simulink subsystem "joystick_to_pwm"  (R2025b)
settings: Solver=VariableStepAuto  StartTime=0.0  StopTime=10.0  RelTol=1e-3
settings Model: Creator=vulcangrip  LastModifiedBy=vulcangrip

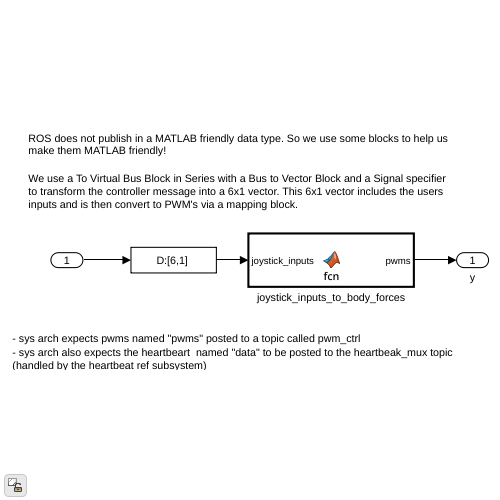
[thumbnail: Simulink's stored preview of the top-level diagram]
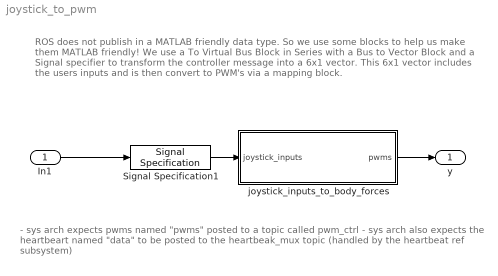
== system joystick_to_pwm ==
  note: - sys arch expects pwms named "pwms" posted to a topic called pwm_ctrl
      | - sys arch also expects the heartbeart  named "data" to be posted to the heartbeak_mux topic (handled by the heartbeat ref subsystem)
  note: ROS does not publish in a MATLAB friendly data type. So we use some blocks to help us make them MATLAB friendly!
      |
      | We use a To Virtual Bus Block in Series with a Bus to Vector Block and a Signal specifier to transform the controller message into a 6x1 vector. This 6x1 vector includes the users inputs and is then convert to PWM's via a mapping block.
  In1 : Inport
  Signal Specification1 : SignalSpecification  Dimensions=[6,1]
  joystick_inputs_to_body_forces : MATLAB Function  TreatAsAtomicUnit=on
  y : Outport
  wires:
  Signal Specification1/1 -> joystick_inputs_to_body_forces/1(joystick_inputs)
  joystick_inputs_to_body_forces/1(pwms) -> y/1
  In1/1 -> Signal Specification1/1

== matlab function joystick_to_pwm/joystick_inputs_to_body_forces ==
  data: pwms output; joystick_inputs input


function pwms = fcn(joystick_inputs)

%Create the mapping here for PWM values.
%Recall that PWM 1-8 correspond to thruster postions which follow,

%pwm of each thruster on the robot
%In left to right:
%f = front / r = rear
%l = left  / r = right
%t = top   / b = bottom
%PWM(1)=pwm_flt
%PWM(2)=pwm_frt
%PWM(3)=pwm_rlt
%PWM(4)=pwm_rrt
%PWM(5)=pwm_flb
%PWM(6)=pwm_frb
%PWM(7)=pwm_rlb
%PWM(8)=pwm_rrb
  
x_joy = joystick_inputs(1);
y_joy = joystick_inputs(2);
rise = joystick_inputs(3);
sink = joystick_inputs(4);
yaw = joystick_inputs(5);
pitch = joystick_inputs(6);


scale = 300;
stop_set = 1500;
max_pwm = 1500+scale;
min_pwm = 1500-scale;

%x_body and y_body mapping
x = y_joy;
y = x_joy;

pwms_vert = stop_set*ones(1,4); %Thrusters 0,1,2,3
pwms_horiz = stop_set*ones(1,4); %Thrusters 4,5,6,7
inversion_mask = [1, -1, 1, -1];

% Rise/Sink
for i = 1:4
    pwms_vert(i) = pwms_vert(i) + (scale*rise - scale*sink) * inversion_mask(i);
end

%Pitch
pwms_vert(1) = pwms_vert(1) - (scale*pitch*inversion_mask(1));
pwms_vert(2) = pwms_vert(2) - (scale*pitch*inversion_mask(2));
pwms_vert(3) = pwms_vert(3) + (scale*pitch*inversion_mask(3));
pwms_vert(4) = pwms_vert(4) + (scale*pitch*inversion_mask(4));

% Forwards:
pwms_horiz(1) = pwms_horiz(1) + scale*x;
pwms_horiz(2) = pwms_horiz(2) - scale*x;
pwms_horiz(3) = pwms_horiz(3) + scale*x;
pwms_horiz(4) = pwms_horiz(4) - scale*x;

% Strafe:
pwms_horiz(1) = pwms_horiz(1) + y*scale;
pwms_horiz(2) = pwms_horiz(2) + y*scale;
pwms_horiz(3) = pwms_horiz(3) - y*scale;
pwms_horiz(4) = pwms_horiz(4) - y*scale;

% Yaw:
pwms_horiz(1) = pwms_horiz(1) + yaw*scale;
pwms_horiz(2) = pwms_horiz(2) + yaw*scale;
pwms_horiz(3) = pwms_horiz(3) + yaw*scale;
pwms_horiz(4) = pwms_horiz(4) + yaw*scale;


for i = 1:4
    if(pwms_horiz(i) > max_pwm)
        pwms_horiz(i) = max_pwm;
    end
    if(pwms_horiz(i) < min_pwm)
        pwms_horiz(i) = min_pwm;
    end
    if(pwms_vert(i) > max_pwm)
        pwms_vert(i) = max_pwm;
    end
    if(pwms_vert(i) < min_pwm)
        pwms_horiz(i) = min_pwm;
    end

end

pwms = int32([pwms_vert,pwms_horiz])';
